simulink subsystem "Liear accleration model"  (R2024a)
settings: Solver=VariableStepAuto  StartTime=0.0  StopTime=10.0  RelTol=1e-3
libraries: autolibshared x6
(part 4 of 4)

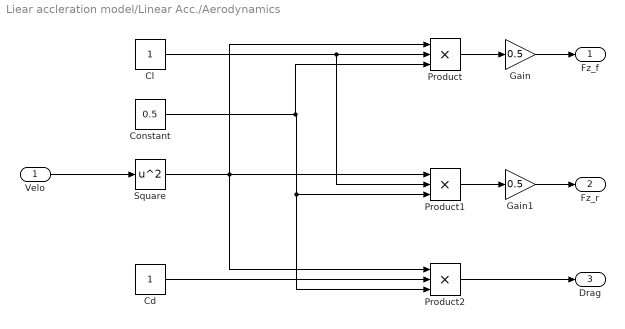
== system Liear accleration model/Linear Acc./Aerodynamics ==
  Velo : Inport
  Cd : Constant
  Cl : Constant
  Constant : Constant  Value=0.5
  Gain : Gain  Gain=0.5
  Gain1 : Gain  Gain=0.5
  Product : Product  Inputs=3
  Product1 : Product  Inputs=3
  Product2 : Product  Inputs=3
  Square : Math  Operator=square
  Fz_f : Outport
  Fz_r : Outport  Port=2
  Drag : Outport  Port=3
  wires:
  Velo/1 -> Square/1
  Product/1 -> Gain/1
  Product1/1 -> Gain1/1
  Product2/1 -> Drag/1
  Gain/1 -> Fz_f/1
  Gain1/1 -> Fz_r/1
  Square/1 -> Product2/1, Product1/1, Product/1
  Cl/1 -> Product1/2, Product/2
  Cd/1 -> Product2/2
  Constant/1 -> Product/3, Product2/3, Product1/3

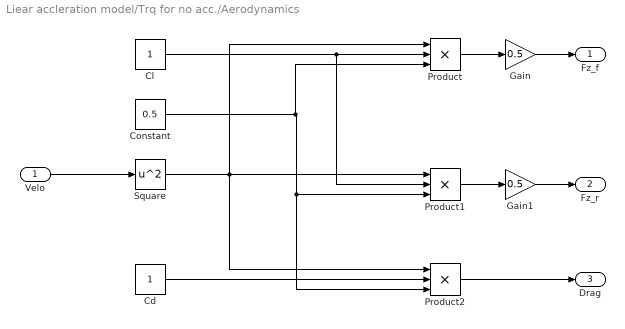
== system Liear accleration model/Trq for no acc./Aerodynamics ==
  Velo : Inport
  Cd : Constant
  Cl : Constant
  Constant : Constant  Value=0.5
  Gain : Gain  Gain=0.5
  Gain1 : Gain  Gain=0.5
  Product : Product  Inputs=3
  Product1 : Product  Inputs=3
  Product2 : Product  Inputs=3
  Square : Math  Operator=square
  Fz_f : Outport
  Fz_r : Outport  Port=2
  Drag : Outport  Port=3
  wires:
  Velo/1 -> Square/1
  Product/1 -> Gain/1
  Product1/1 -> Gain1/1
  Product2/1 -> Drag/1
  Gain/1 -> Fz_f/1
  Gain1/1 -> Fz_r/1
  Square/1 -> Product2/1, Product1/1, Product/1
  Cl/1 -> Product1/2, Product/2
  Cd/1 -> Product2/2
  Constant/1 -> Product/3, Product2/3, Product1/3
